simulink model "prob5_week1"  (R2020b)
settings: Solver=VariableStepAuto  StartTime=0.0  StopTime=10.0  RelTol=1e-3
settings Model: Creator=Pulkit Khandelwal  LastModifiedBy=Pulkit Khandelwal

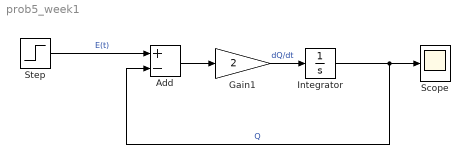
== system prob5_week1 ==
  Add : Sum  Inputs=+-
  Gain1 : Gain  Gain=2
  Integrator : Integrator
  Scope : Scope
  Step : Step  Before=1  After=5  SampleTime=0
  wires:
  Integrator/1 -> Add/2, Scope/1  "Q"
  Gain1/1 -> Integrator/1  "dQ/dt"
  Step/1 -> Add/1  "E(t)"
  Add/1 -> Gain1/1
